simulink model "Project"  (R2024b)
settings: Solver=FixedStepAuto  StartTime=0.0  StopTime=Inf  RelTol=1e-3  EnableMultiTasking=on
libraries: stm32f4xxblockslib x10, stm32blockslib x2
settings Model: STM32="{\"UARTRead\":[{\"ID\":\"ProvaStringaUART:41\"},{\"ID\":\"Progetto_Embedded_Gruppo11:41\"}],\"UARTWrite\":[{\"ID\":\"ProvaStringaUART:43\"},{\"ID\":\"Progetto_Embedded_Gruppo11:43\"}],\"DigitalPortRead\":[{\"ID\":\"ProvaStringaUART:48\"},{\"ID\":\"ProvaStringaUART:49\"},{\"ID\":\"ProvaStringaUART:51\"},{\"ID\":\"ProvaStringaUART:52\"},{\"ID\":\"Progetto_Embedded_Gruppo11:52\"},{\"ID\":\"Progetto_Embedded_Gruppo11:51\"},{\"ID\":\"Progetto_Embedded_Gruppo11:49\"},{\"ID\":\"Progetto_Embedded_Gruppo11:48\"}],\"DigitalPortWrite\":[{\"ID\":\"ProvaStringaUART:50\"},{\"ID\":\"ProvaStringaUART:74\"},{\"ID\":\"Progetto_Embedded_Gruppo11:74\"},{\"ID\":\"Progetto_Embedded_Gruppo11:50\"}],\"PWMOutput\":[{\"ID\":\"ProvaStringaUART:58\"},{\"ID\":\"ProvaStringaUART:68\"},{\"ID\":\"ProvaStringaUART:69\"},{\"ID\":\"ProvaStringaUART:70\"},{\"ID\":\"Progetto_Embedded_Gruppo11:70\"},{\"ID\":\"Progetto_Embedded_Gruppo11:69\"},{\"ID\":\"Progetto_Embedded_Gruppo11:68\"},{\"ID\":\"Progetto_Embedded_Gruppo11:58\"}]}"  PacingRate=0.100000  Creator=114973  LastModifiedBy=feder
settings OptimizationCC: DefaultParameterBehavior=Inlined  EnhancedBackFolding=on  PassReuseOutputArgsAs=Individual arguments  ZeroExternalMemoryAtStartup=off  ZeroInternalMemoryAtStartup=off  MaxStackSize=512  OptimizeBlockOrder=speed  DifferentSizesBufferReuse=on  OptimizationCustomize=off  EfficientTunableParamExpr=on
settings DebuggingCC: ParameterTunabilityLossMsg=error
settings HardwareCC: ProdBitPerPointer=32  ProdBitPerSizeT=32  ProdBitPerPtrDiffT=32  ProdLargestAtomicInteger=Long  ProdLargestAtomicFloat=Double  ProdWordSize=32  ProdHWDeviceType=ARM Compatible->ARM Cortex-M
settings RTWCC: Description=Embedded Coder  SystemTargetFile=ert.tlc  HardwareBoard=STM32G4xx Based  TemplateMakefile=ert_default_tmf  Toolchain=GNU Tools for ARM Embedded Processors
settings CodeAppCC: ForceParamTrailComments=on  IgnoreCustomStorageClasses=off  OperatorAnnotations=on  SimulinkDataObjDesc=on  SFDataObjDesc=on  InsertBlockDesc=on
settings ERTTargetCC: TargetLangStandard=C99 (ISO)  CodeReplacementLibrary=ARM Cortex-M  SupportVariableSizeSignals=on  ExtModeTransport=3  ExtModeStaticAlloc=on  ExtModeStaticAllocSize=2048  ExtModeMexFile=ext_xcp  ExtModeIntrfLevel=Level2 - Open

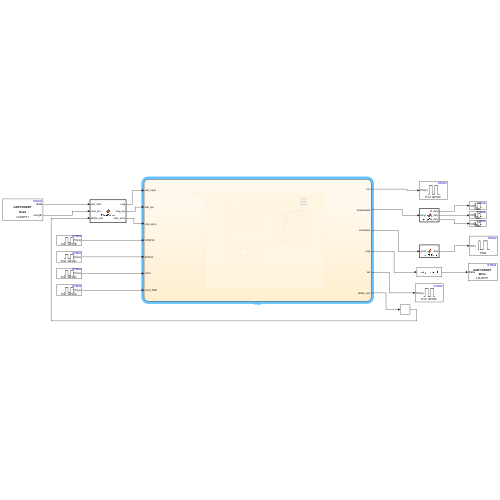
[thumbnail: Simulink's stored preview of the top-level diagram]
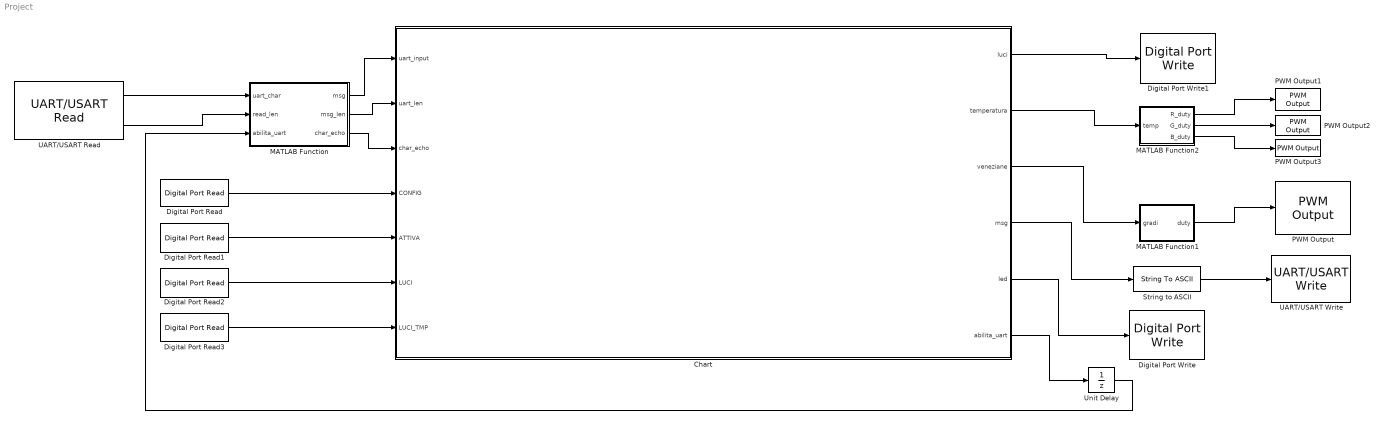
== system Project ==
  Chart : Stateflow chart  TreatAsAtomicUnit=on
  Digital Port Read : stm32f4xxblockslib/Digital Port Read  PortName=GPIOB  PinNumber=[0]  ReadOperation=on  IOAsArray=on  SampleTime=-1  EnableSimPort=off  hoistedMaskSrc=ECSoC/ECSimCodegen/Digital Port Read
  Digital Port Read1 : stm32f4xxblockslib/Digital Port Read  PortName=GPIOC  PinNumber=[13]  ReadOperation=on  IOAsArray=on  SampleTime=-1  EnableSimPort=off  hoistedMaskSrc=ECSoC/ECSimCodegen/Digital Port Read
  Digital Port Read2 : stm32f4xxblockslib/Digital Port Read  PortName=GPIOC  PinNumber=[10]  ReadOperation=on  IOAsArray=on  SampleTime=-1  EnableSimPort=off  hoistedMaskSrc=ECSoC/ECSimCodegen/Digital Port Read
  Digital Port Read3 : stm32f4xxblockslib/Digital Port Read  PortName=GPIOA  PinNumber=[15]  ReadOperation=on  IOAsArray=on  SampleTime=-1  EnableSimPort=off  hoistedMaskSrc=ECSoC/ECSimCodegen/Digital Port Read
  Digital Port Write : stm32f4xxblockslib/Digital Port Write  PortName=GPIOA  PinNumber=[5]  ReadOperation=off  IOAsArray=on  EnableSimPort=off  hoistedMaskSrc=ECSoC/ECSimCodegen/Digital Port Write
  Digital Port Write1 : stm32f4xxblockslib/Digital Port Write  PortName=GPIOC  PinNumber=[2]  ReadOperation=off  IOAsArray=on  EnableSimPort=off  hoistedMaskSrc=ECSoC/ECSimCodegen/Digital Port Write
  MATLAB Function : MATLAB Function  TreatAsAtomicUnit=on
  MATLAB Function1 : MATLAB Function  TreatAsAtomicUnit=on
  MATLAB Function2 : MATLAB Function  TreatAsAtomicUnit=on
  PWM Output : stm32f4xxblockslib/PWM Output  TimerModule=TIM4  DutycycleUnits=Percentage  EnableChannel1=on  EnableChannel2=off  EnableChannel3=off  EnableChannel4=off  EnableCounterInput=off  EnableMainOutputInput=off  EnableFrequencyInput=off  SetRCAfterCE=off  OutputDirection=off  OutputMainOutputEnableStatus=off  SampleTime=0.1  EnableSimPort=off  EnableUpdateEvent=off  EnableCaptureCompare1Event=off  EnableCaptureCompare2Event=off  EnableCaptureCompare3Event=off  EnableCaptureCompare4Event=off  EnableTriggerEvent=off  EnableBreakEvent=off  ProcessorFamily=STM32F4  hoistedMaskSrc=ECSoC/ECSimCodegen/PWM Output
  PWM Output1 : stm32f4xxblockslib/PWM Output  TimerModule=TIM3  DutycycleUnits=Percentage  EnableChannel1=on  EnableChannel2=off  EnableChannel3=off  EnableChannel4=off  EnableCounterInput=off  EnableMainOutputInput=off  EnableFrequencyInput=off  SetRCAfterCE=off  OutputDirection=off  OutputMainOutputEnableStatus=off  SampleTime=0.1  EnableSimPort=off  EnableUpdateEvent=off  EnableCaptureCompare1Event=off  EnableCaptureCompare2Event=off  EnableCaptureCompare3Event=off  EnableCaptureCompare4Event=off  EnableTriggerEvent=off  EnableBreakEvent=off  ProcessorFamily=STM32F4  hoistedMaskSrc=ECSoC/ECSimCodegen/PWM Output
  PWM Output2 : stm32f4xxblockslib/PWM Output  TimerModule=TIM3  DutycycleUnits=Percentage  EnableChannel1=off  EnableChannel2=on  EnableChannel3=off  EnableChannel4=off  EnableCounterInput=off  EnableMainOutputInput=off  EnableFrequencyInput=off  SetRCAfterCE=off  OutputDirection=off  OutputMainOutputEnableStatus=off  SampleTime=0.1  EnableSimPort=off  EnableUpdateEvent=off  EnableCaptureCompare1Event=off  EnableCaptureCompare2Event=off  EnableCaptureCompare3Event=off  EnableCaptureCompare4Event=off  EnableTriggerEvent=off  EnableBreakEvent=off  ProcessorFamily=STM32F4  hoistedMaskSrc=ECSoC/ECSimCodegen/PWM Output
  PWM Output3 : stm32f4xxblockslib/PWM Output  TimerModule=TIM3  DutycycleUnits=Percentage  EnableChannel1=off  EnableChannel2=off  EnableChannel3=off  EnableChannel4=on  EnableCounterInput=off  EnableMainOutputInput=off  EnableFrequencyInput=off  SetRCAfterCE=off  OutputDirection=off  OutputMainOutputEnableStatus=off  SampleTime=0.1  EnableSimPort=off  EnableUpdateEvent=off  EnableCaptureCompare1Event=off  EnableCaptureCompare2Event=off  EnableCaptureCompare3Event=off  EnableCaptureCompare4Event=off  EnableTriggerEvent=off  EnableBreakEvent=off  ProcessorFamily=STM32F4  hoistedMaskSrc=ECSoC/ECSimCodegen/PWM Output
  String to ASCII : StringToASCII  OutputVectorSize=130
  UART/USART Read : stm32blockslib/UART//USART Read  UARTModule=LPUART1  DataType=uint8  DataLength=1  BlockingMode=off  BlockingTimeout=0.1  OutputLength=on  OutputStatus=off  SampleTime=-1
      settings: LibrarySourceBlock=stm32g4xxblockslib/UART//USART Read
  UART/USART Write : stm32blockslib/UART//USART Write  UARTModule=LPUART1  LengthOfDataToSend=off  BlockingMode=off  BlockingTimeout=0.1  OutputStatus=off
      settings: LibrarySourceBlock=stm32g4xxblockslib/UART//USART Write
  Unit Delay : UnitDelay  SampleTime=-1  HasFrameUpgradeWarning=on
  wires:
  UART/USART Read/1 -> MATLAB Function/1(uart_char)
  MATLAB Function/1(msg) -> Chart/1(uart_input)
  Chart/4(msg) -> String to ASCII/1
  String to ASCII/1 -> UART/USART Write/1
  MATLAB Function/3(char_echo) -> Chart/3(char_echo)
  UART/USART Read/2 -> MATLAB Function/2(read_len)
  MATLAB Function/2(msg_len) -> Chart/2(uart_len)
  Digital Port Read/1 -> Chart/4(CONFIG)
  Digital Port Read1/1 -> Chart/5(ATTIVA)
  Chart/5(led) -> Digital Port Write/1
  Digital Port Read3/1 -> Chart/7(LUCI_TMP)
  Digital Port Read2/1 -> Chart/6(LUCI)
  Chart/3(veneziane) -> MATLAB Function1/1(gradi)
  MATLAB Function1/1(duty) -> PWM Output/1
  Chart/2(temperatura) -> MATLAB Function2/1(temp)
  MATLAB Function2/1(R_duty) -> PWM Output1/1
  MATLAB Function2/2(G_duty) -> PWM Output2/1
  MATLAB Function2/3(B_duty) -> PWM Output3/1
  Chart/1(luci) -> Digital Port Write1/1
  Chart/6(abilita_uart) -> Unit Delay/1
  Unit Delay/1 -> MATLAB Function/3(abilita_uart)

== matlab function Project/MATLAB Function1 ==
  data: gradi input; duty output
function duty = gradiToDuty(gradi)
%#codegen

% Mappa i gradi [0:20:180] in duty [%] da 12.5 a 2.5 (servo inverso)
switch gradi
    case 0
        duty = 2.50;
    case 20
        duty = 3.62;
    case 40
        duty = 4.73;
    case 60
        duty = 5.84;
    case 80
        duty = 6.95;
    case 100
        duty = 8.06;
    case 120
        duty = 9.17;
    case 140
        duty = 10.28;
    case 160
        duty = 11.39;
    case 180
        duty = 12.50;
    otherwise
        duty = 2.50;  % errore o valore fuori range
end

== matlab function Project/MATLAB Function ==
  data: uart_char input; msg output; msg_len output; char_echo output; read_len input; abilita_uart input
function [msg, msg_len, char_echo] = CharBuffer(uart_char, read_len, abilita_uart)
%#codegen

% persistent per mantenere buffer e indice precedenti ad ogni nuovo
% carattere inserito
persistent buffer idx

% inizializzo il buffer con dimensione 50 byte solo al primo avvio.
if isempty(buffer)
    buffer = zeros(1, 50, 'uint8');  % massimo 50 caratteri
    idx = 1; %indici partono da 1
end

%Nel sistema l'uart_input viene già dato come stringa.

msg = "";         % messaggio completo, da valutare dopo invio
msg_len = 0;      % lunghezza messaggio, utile per effettuare controlli ed evitare loop con lo stato di errore
char_echo = "";   % singolo carattere ricevuto da stampare subito

if read_len > 0 && abilita_uart==1 %se sto leggendo qualcosa da UART
    % Echo del carattere se non è invio
    if uart_char ~= 10 && uart_char ~= 13
        char_echo = string(char(uart_char));   %byte si converte in char e poi in string
    end

    % Se è INVIO (enter)
    if uart_char == 10 || uart_char == 13
        if idx > 1                              % se non ho inserito solo \n o solo \r
            raw = char(buffer(1:idx-1));        % solo le lettere inserite, scartando carattere \n finale
            cleaned = strtrim(string(raw));     % rimuove spazi, \n, \r
            msg = cleaned;                      % setto cleaned come messaggio da dare in input
            msg_len = strlength(cleaned);       % prendo la sua lunghezza da dare in input
        end
        buffer(:) = 0;                          %resetto buffer (già allocato all'avvio)
        idx = 1;                                %resetto indice
    elseif uart_char == 8 || uart_char == 127  % ASCII per backspace
    if idx > 1
        idx = idx - 1;
        buffer(idx) = 0;  % Cancella ultimo carattere
    end


    elseif idx <= 50
            buffer(idx) = uart_char;
            idx = idx + 1;
        
     end
   else                                            %se non sto leggendo nulla da terminale
       char_echo = "";                             % stampo il vuoto per evitare ripetizioni dell'ultimo carattere digitato (problema visivo e logico)
end

== stateflow chart Project/Chart ==
  state STATO_ATTIVO
    en:
    if stato==1
    luci = oldLuci;
    veneziane = oldVeneziane;
    temperatura = oldTemperatura;
    temporizzazione = oldTemporizzazione;
    end
    state SISTEMA [parallel]
      settings: executionOrder=1
      state CONFIGURAZIONE
        en:
        abilita_uart=1;
        state ERROR
          en: msg = string(char(eol)) + ...
          "Input non valido! Riprova." + string(char(eol));
          ex: msg = "";
        state SELEZIONE_MOD
          en: msg = string(char(eol)) + ...
          "Digita cosa vuoi configurare. Inserisci luci, temperatura, veneziane oppure conferma." + ...
          string(char(eol));
          du: msg = "";
          if uart_len == 0 && strlength(char_echo) > 0
          msg = char_echo;
          end
        state CONFERMA
          en:
          if oldLuci == 255 || oldTemporizzazione == 255 || oldTemperatura == 255 || oldVeneziane == 255
          msg = string(char(eol)) + ...
          "Occorre inserire una configurazione valida per ogni funzione." + string(char(eol));
          stato = 0;
          else
          msg = string(char(eol)) + "Configurazione salvata." + string(char(eol));
          stato = 1;
          end
          ex:
          msg = "";
        state SET_TEMPERATURA
          en:
          msg=string(char(eol)) + ...
          "Inserisci configurazione per la temperatura. Digita un valore intero tra 16 e 30" + string(char(eol));
          du:
          msg = "";
          if uart_len == 0 && strlength(char_echo) > 0
          msg = char_echo;
          end
          if TemperaturaIsValid(uart_input)
          temp = sscanf(char(uart_input), '%d');
          converted_input = uint8(temp(1));
          oldTemperatura = converted_input;
          end
        state SET_VENEZIANE
          en: msg= string(char(eol)) + ...
          "Inserisci configurazione per le veneziane. Digita un valore tra i seguenti: 0, 20, 40, 60, 80, 100, 120, 140, 160, 180." + ...
          string(char(eol));
          du: msg= "";
          if uart_len == 0 && strlength(char_echo) > 0
          msg = char_echo;
          end
          if VenezianeIsValid(uart_input)
          temp = sscanf(char(uart_input), '%d');
          converted_input = uint8(temp(1));
          oldVeneziane = converted_input;
          end
        state SET_LUCE
          en:
          msg = string(char(eol)) + ...
          "Inserisci configurazione per le luci. Digita ON oppure OFF" + ...
          string(char(eol));
          du:
          msg = "";
          if uart_len == 0 && strlength(char_echo) > 0
          msg = char_echo;
          end
          if strcmp(uart_input,"ON")
          oldLuci = ON;
          end
          if strcmp(uart_input,"OFF")
          oldLuci = OFF;
          end
        state SET_TEMP
          en:
          msg = string(char(eol)) + ...
          "Inserisci 0 per disattivare la temporizzazione oppure un valore tra 5 e 30" + ...
          string(char(eol));
          du:
          msg = "";
          if uart_len == 0 && strlength(char_echo) > 0
          msg = char_echo;
          end
          if TemporizzazioneIsValid(uart_input)
          temp = sscanf(char(uart_input), '%d');
          converted_input = uint8(temp(1));
          oldTemporizzazione = converted_input;
          end
        ERROR -> SELEZIONE_MOD [order 1] : [error == "menu"]
        (default) -> SELEZIONE_MOD
        SELEZIONE_MOD -> ERROR [order 5] : [uart_len > 0]{error = "menu"}
        ERROR -> SET_TEMP [order 3] : [error == "tempo"]
        SET_TEMP -> ERROR [order 1] : [uart_len > 0 && ~strcmp(uart_input, "exit") && ~TemporizzazioneIsValid(uart_input)]{error="tempo"}
        SET_LUCE -> ERROR [order 1] : [uart_len > 0 && ~strcmp(uart_input, "exit") && ~strcmp(uart_input, "ON") && ~strcmp(uart_input, "OFF")]{error = "luci"}
        ERROR -> SET_LUCE [order 2] : [error == "luci"]
        SET_TEMPERATURA -> ERROR [order 1] : [uart_len > 0 && ~strcmp(uart_input, "exit") && ~TemperaturaIsValid(uart_input)]{error="temperatura"}
        ERROR -> SET_TEMPERATURA [order 5] : [error == "temperatura"]
        ERROR -> SET_VENEZIANE [order 4] : [error == "veneziane"]
        SET_VENEZIANE -> ERROR [order 1] : [uart_len > 0 && ~strcmp(uart_input, "exit") && ~VenezianeIsValid(uart_input)]{error = "veneziane"}
        SET_TEMP -> SELEZIONE_MOD [order 2] : [change(oldTemporizzazione) || (uart_len > 0 && strcmp(uart_input, "exit"))]
        SET_LUCE -> SELEZIONE_MOD [order 3] : [uart_len > 0 && strcmp(uart_input, "exit")]
        SELEZIONE_MOD -> SET_LUCE [order 1] : [uart_len > 0 && strcmp(uart_input, "luci")]
        SET_VENEZIANE -> SELEZIONE_MOD [order 2] : [change(oldVeneziane) || (uart_len > 0 && strcmp(uart_input, "exit"))]
        SELEZIONE_MOD -> SET_VENEZIANE [order 2] : [uart_len > 0 && strcmp(uart_input, "veneziane")]
        SELEZIONE_MOD -> SET_TEMPERATURA [order 3] : [uart_len > 0 && strcmp(uart_input, "temperatura")]
        SET_TEMPERATURA -> SELEZIONE_MOD [order 2] : [change(oldTemperatura) || (uart_len > 0 && strcmp(uart_input, "exit"))]
        CONFERMA -> SELEZIONE_MOD [order 1] : [stato == 0]
        SELEZIONE_MOD -> CONFERMA [order 4] : [uart_len > 0 && strcmp(uart_input,"conferma")]
        SET_LUCE -> SET_TEMP [order 2] : [change(oldLuci)]
      state OPERATIVO
        en:
        abilita_uart=0;
        state LUCI [parallel]
          settings: executionOrder=2
          state ON
            en: luci = ON;
          state OFF
            en: luci = OFF
          state TEMP
            en: luci = ON
          (default) -> (junction 267)
          (junction 267) -> OFF [order 2]
          (junction 267) -> ON [order 1] : [luci == ON]
          OFF -> ON [order 2] : [LUCI == Pressed]
          ON -> OFF [order 2] : [LUCI == Pressed]
          ON -> TEMP [order 1] : [temporizzazione ~= 0 && LUCI_TMP == Pressed]
          TEMP -> OFF : after(temporizzazione, sec)
          OFF -> TEMP [order 1] : [temporizzazione ~= 0 && LUCI_TMP == Pressed]
        state TRASMISSIONE_STATO [parallel]
          settings: executionOrder=1
          note: Stampa dello stato corrente del dispositivo ogni 10 secondi
          state NOTIFICA
            en:
            msg = string(char(eol)) + ...
            "Luci: " + string(luci) + ...
            ", Temporizzazione: " + string(temporizzazione) + ...
            ", Veneziane: " + string(veneziane) + ...
            ", Temperatura: " + string(temperatura) + ...
            string(char(eol));
            du:
            msg = "";
          (default) -> NOTIFICA
          NOTIFICA -> NOTIFICA : after(10,sec)
      (junction 234) -> CONFIGURAZIONE [order 2]
      (default) -> (junction 234)
      (junction 234) -> OPERATIVO [order 1] : [stato == 1]
      OPERATIVO -> CONFIGURAZIONE : [CONFIG == Pressed]
      CONFIGURAZIONE -> OPERATIVO : [CONFIG == Pressed && stato == 1]
      CONFERMA -> OPERATIVO [order 2] : [stato == 1]{luci = oldLuci; veneziane = oldVeneziane; temperatura = oldTemperatura; temporizzazione = oldTemporizzazione;}
    state LED [parallel]
      settings: executionOrder=2
      state LED_ON
        en:
        led=ON;
      state LED_OFF
        en:
        led=OFF;
      (default) -> LED_ON
      LED_ON -> LED_OFF : after(0.5, sec)
      LED_OFF -> LED_ON : after(0.5, sec)
  state STATO_DISATTIVO
    en: luci = OFF;
    veneziane = 0;
    temperatura = 16;
    temporizzazione = OFF;
    led = OFF;
    msg = char(27) + "[2J" + char(27) + "[H";  % pulisci terminale
    abilita_uart=0;
  (default) -> STATO_DISATTIVO
  STATO_DISATTIVO -> STATO_ATTIVO : [ATTIVA == Pressed]
  STATO_ATTIVO -> STATO_DISATTIVO : [ATTIVA == Pressed]
  data: uart_input function_input; isValid function_output; uart_input function_input; isValid function_output; uart_input function_input; isValid function_output; OFF constant uint8 =0; luci output uint8; temperatura output uint8; veneziane output uint8; oldLuci local uint8 =255; oldTemperatura local uint8 =255; oldTemporizzazione local uint8 =255; oldVeneziane local uint8 =255; ON constant uint8 =1; uart_input input string; uart_len input; msg output string; error local string; temp local size=[10 1]; converted_input local uint8 size=1 =0; stato local =0; char_echo input; eol constant uint8 size=[1 2] =[13 10]; CONFIG input; Pressed constant double =1; ATTIVA input; led output; LUCI input; LUCI_TMP input; temporizzazione local uint8; abilita_uart output =0
  function isValid = VenezianeIsValid(uart_input):
    | function isValid = VenezianeIsValid(uart_input)
    | % Restituisce true se l'input È valido
    | 
    |     valid_values = {'0', '20', '40', '60', '80', ...
    |                     '100', '120', '140', '160', '180'};
    |     isValid = any(strcmp(uart_input, valid_values));
    | end
  function isValid = TemporizzazioneIsValid(uart_input):
    | function isValid = TemporizzazioneIsValid(uart_input)
    | % Restituisce true se l'input è valido per la temporizzazione
    | % Valori validi: '0' oppure da '5' a '30'
    | 
    |     valid_values = {'0', '5', '6', '7', '8', '9', ...
    |                     '10', '11', '12', '13', '14', '15', '16', '17', '18', '19', ...
    |                     '20', '21', '22', '23', '24', '25', '26', '27', '28', '29', '30'};
    |                 
    |     isValid = any(strcmp(uart_input, valid_values));
    | end
  function isValid = TemperaturaIsValid(uart_input):
    | function isValid = TemperaturaIsValid(uart_input)
    | % Restituisce true se l'input è valido per la temperatura
    | % Valori validi: da '16' a '30'
    | 
    |     valid_values = {'16', '17', '18', '19', ...
    |                     '20', '21', '22', '23', '24', '25', ...
    |                     '26', '27', '28', '29', '30'};
    |                 
    |     isValid = any(strcmp(uart_input, valid_values));
    | end

== matlab function Project/MATLAB Function2 ==
  data: temp input; R_duty output; G_duty output; B_duty output
function [R_duty, G_duty, B_duty] = mapColor(temp)
    % Mappa temperatura a valori RGB (0–1)

    if temp >= 16 && temp <= 18
        R = 0; G = 0; B = 1;        % Blu
    elseif temp >= 19 && temp <= 21
        R = 0.5; G = 0; B = 0.5;    % Viola
    elseif temp >= 22 && temp <= 24
        R = 1; G = 0.5; B = 0;        % Giallo
    elseif temp >= 25 && temp <= 27
        R = 1; G = 0.2; B = 0;      % Arancione
    else temp >= 28 && temp <= 30
        R = 1; G = 0; B = 0;        % Rosso
    end

    % Conversione a duty cycle (%)
    R_duty = R * 100;
    G_duty = G * 100;
    B_duty = B * 100;

end
